simulink model "task1"  (R2022a)
settings: Solver=FixedStepAuto  StartTime=0.0  StopTime=1  FixedStep=10e-4  RelTol=1e-3
undefined symbols (not defined in the file or in its folder): den, K, K1
settings Model: Creator=mikol  LastModifiedBy=mikol

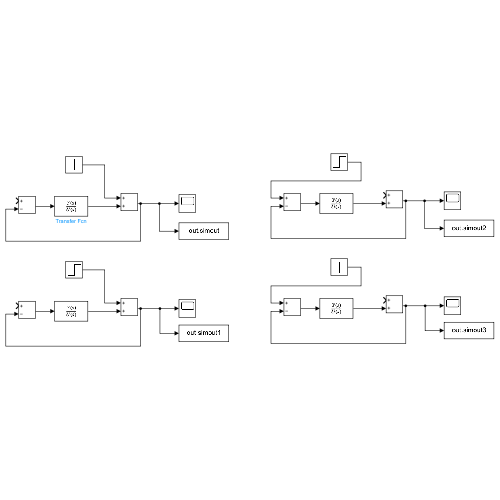
[thumbnail: Simulink's stored preview of the top-level diagram]
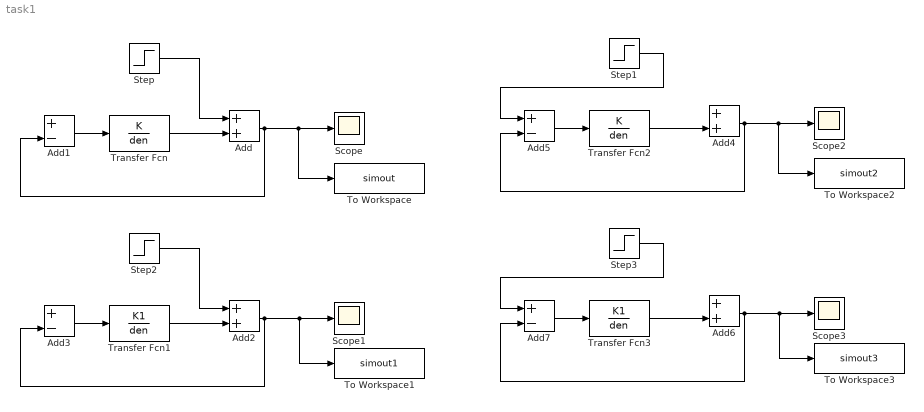
== system task1 ==
  Add{,2,4,6} (4 alike) : Sum
  Add{1,3,5,7} (4 alike) : Sum  Inputs=+-
  Scope{,1..3} (4 alike) : Scope
  Step{,1..3} (4 alike) : Step  Time=0  SampleTime=0
  To Workspace : ToWorkspace  VariableName=simout  SampleTime=-1
      settings: Save2DSignal=2-D array (concatenate along first dimension)
  To Workspace1 : ToWorkspace  VariableName=simout1  SampleTime=-1
      settings: Save2DSignal=2-D array (concatenate along first dimension)
  To Workspace2 : ToWorkspace  VariableName=simout2  SampleTime=-1
      settings: Save2DSignal=2-D array (concatenate along first dimension)
  To Workspace3 : ToWorkspace  VariableName=simout3  SampleTime=-1
      settings: Save2DSignal=2-D array (concatenate along first dimension)
  Transfer Fcn : TransferFcn  Numerator=K  Denominator=den
  Transfer Fcn1 : TransferFcn  Numerator=K1  Denominator=den
  Transfer Fcn2 : TransferFcn  Numerator=K  Denominator=den
  Transfer Fcn3 : TransferFcn  Numerator=K1  Denominator=den
  wires:
  Add/1 -> Add1/2, To Workspace/1, Scope/1
  Transfer Fcn/1 -> Add/2
  Step/1 -> Add/1
  Add1/1 -> Transfer Fcn/1
  Transfer Fcn1/1 -> Add2/2
  Step2/1 -> Add2/1
  Add2/1 -> Add3/2, To Workspace1/1, Scope1/1
  Add3/1 -> Transfer Fcn1/1
  Add6/1 -> Add7/2, To Workspace3/1, Scope3/1
  Add7/1 -> Transfer Fcn3/1
  Transfer Fcn3/1 -> Add6/2
  Transfer Fcn2/1 -> Add4/2
  Add4/1 -> Add5/2, To Workspace2/1, Scope2/1
  Add5/1 -> Transfer Fcn2/1
  Step1/1 -> Add5/1
  Step3/1 -> Add7/1
